simulink model "Furuta_Control"  (R2017a)
settings: Solver=FixedStepAuto  StartTime=0.0  StopTime=10  FixedStep=Ts  RelTol=1e-3
PreLoadFcn:
  | %myBusDef
StartFcn:
  | % Full path to the block
  | %blk = 'Furuta_Control/Bus Creator';
  | 
  | % Attach the event listener
  | %h = add_exec_event_listener(blk, ...
  | %         'PostOutputs', @displayBusdata);
values from neighbouring files (symbols this model uses):
  alpha = J + (M+m1/3+m2)*L1^2    (= 0.00399809399506)    [Furuta_Constants.m]
  beta = (M + m2/3)*L2^2    (= 0.000696322666667)    [Furuta_Constants.m]
  dtDisc = 0.01    [Furuta_Constants.m]
  gamma = (M + m2/2)*L2*L1    (= 0.0006835647)    [Furuta_Constants.m]
  initial_state = pi+15*pi/180    (= 3.40339204139)    [Furuta_Constants.m]
  K = place(Ap,Bp,[-7 -5 -4+4j -4-4j])    [Furuta_Constants.m]
  kb = 2*zeta*omega_n*J    (= 0.000479399222688)    [Furuta_Constants.m]
  ke = 0.182    [Furuta_Constants.m]
  Re = 14.5    [Furuta_Constants.m]
  sigma = (M + m2/2)*g*L2    (= 0.07018074)    [Furuta_Constants.m]
  Ts = 0.001    [Furuta_Constants.m]
libraries: simulink_extras x1, dspinverses x1, sharedTrackingLibrary x1
settings Model: Creator=Marcelo  LastModifiedBy=felip
settings SolverCC: ZeroCrossControl=DisableAll
settings DebuggingCC: ParameterOverflowMsg=warning  BusObjectLabelMismatch=error
settings ModelReferenceCC: ModelReferenceMinAlgLoopOccurrences=on
settings ConfigComp: PLC_TargetIDE=codesys23  PLC_GenerateReport=off

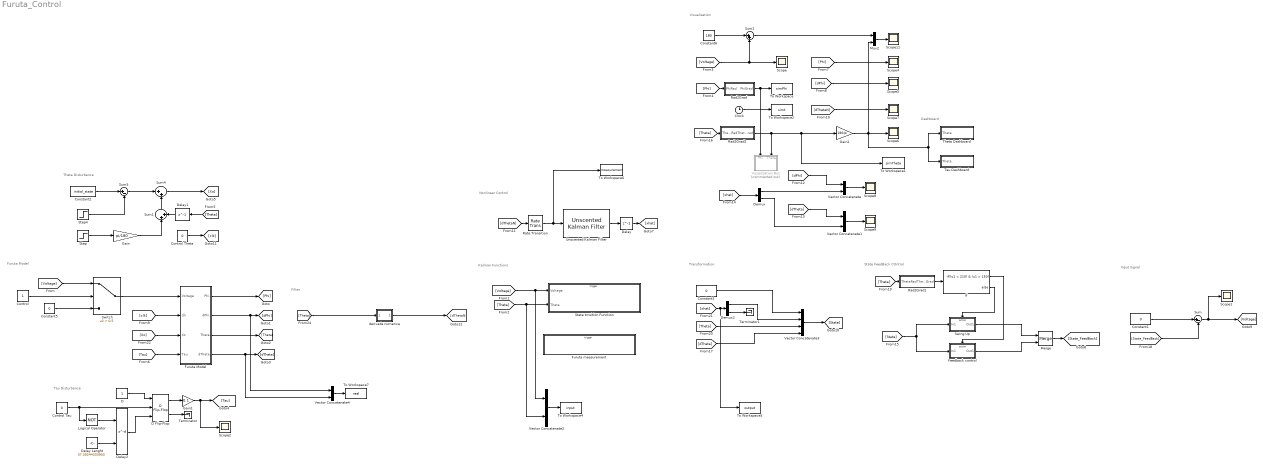
== system Furuta_Control ==
  note: Filter
  note: Tau Disturbance
  note: Dashboard
  note: Theta Disturbance
  note: Transformation
  note: State FeedBack COntrol
  note: Input Signal
  note: Furuta Model
  note: Visualisation
  note: Kalman Functions
  note: Nonlinear Control
  Clock : Clock
  Constant1 : Constant  Value=0
  Constant2 : Constant  Value=initial_state
  Constant3 : Constant  Value=0
  Constant5 : Constant  Value=0
  Constant6 : Constant  Value=180
  Control : Constant
  "Control Tau " : Constant  Value=0  OutDataTypeStr=boolean
  Control Theta : Constant  Value=0
  D : Constant  OutDataTypeStr=boolean
  D Flip-Flop : simulink_extras/Flip Flops/D Flip-Flop
      settings: SourceProductName=Simulink
  Delay : Delay  DelayLength=1  InitialCondition=0
  Delay Lenght : Constant  Value=37.39244333903
  Delay1 : Delay  DelayLength=1
  Delay2 : Delay  DelayLengthSource=Input port
      settings: InputPortMap=u0,p1
  Demux : Demux  Outputs=2
  Demux2 : Demux  Outputs=2
  Feedback control : Subsystem  TreatAsAtomicUnit=on
  "Furuta Model " : Subsystem
  "Furuta measurement " : Subsystem  TreatAsAtomicUnit=on
  Gain : Gain  Gain=pi/180
  Gain1 : Gain  Gain=0.1
  Gain2 : Gain  Gain=180/pi
  If : If  IfExpression=(u1 < 210) & (u1 > 150)
  Logical Operator : Logic  Operator=NOT  AllPortsSameDT=off  OutDataTypeStr=boolean
  Merge : Merge
  Mux2 : Mux  Inputs=2
  Rad2Grad : Subsystem
  Rad2Grad1 : Subsystem
  Rad2Grad2 : Subsystem
  Rate Transition : RateTransition  OutPortSampleTimeOpt=Inherit  OutPortSampleTime=Ts
  Scope{,1..2,4..9,11} (10 alike) : Scope
  "State trnsition Function " : Subsystem  TreatAsAtomicUnit=on
  Step : Step  After=-13.91193695068  SampleTime=0
  Step4 : Step  Time=0.5  After=initial_state  SampleTime=0
  Sum : Sum  Inputs=|+-
  Sum1 : Sum  Inputs=|++
  Sum2 : Sum  Inputs=|++
  Sum4 : Sum  Inputs=|++
  Sum5 : Sum  Inputs=|+-
  Swing Up : Subsystem  TreatAsAtomicUnit=on
  Switch : Switch  Criteria=u2 > Threshold  Threshold=0.5
  Tau Dashboard : Subsystem
  Terminator : Terminator
  Terminator1 : Terminator
  Theta Dashboard : Subsystem
  To Workspace : ToWorkspace  VariableName=simPhi  SampleTime=-1
      settings: Save2DSignal=2-D array (concatenate along first dimension)
  To Workspace1 : ToWorkspace  VariableName=simTheta  SampleTime=-1
      settings: Save2DSignal=2-D array (concatenate along first dimension)
  To Workspace2 : ToWorkspace  VariableName=simt  SampleTime=-1
      settings: Save2DSignal=2-D array (concatenate along first dimension)
  To Workspace4 : ToWorkspace  VariableName=input  SampleTime=-1
      settings: Save2DSignal=2-D array (concatenate along first dimension)
  To Workspace5 : ToWorkspace  VariableName=output  SampleTime=-1
      settings: Save2DSignal=2-D array (concatenate along first dimension)
  To Workspace6 : ToWorkspace  VariableName=measurement  SampleTime=-1
      settings: Save2DSignal=2-D array (concatenate along first dimension)
  To Workspace7 : ToWorkspace  VariableName=real  SampleTime=-1
      settings: Save2DSignal=2-D array (concatenate along first dimension)
  Unscented Kalman Filter : sharedTrackingLibrary/Unscented Kalman Filter  StateTransitionFcn=Furuta_State_Transition  HasAdditiveProcessNoise=Additive  ProcessNoise=diag([2e-8,2e-8])  HasTimeVaryingProcessNoise=off  HasStateTransitionFcnExtraArgument=0  InitialState=[0;0]  InitialStateCovariance=diag([0.001,0.001])  Alpha=1  Beta=2  Kappa=0  MeasurementFcn1=Furuta_Measurement  HasMeasurementEnablePort1=off  HasAdditiveMeasurementNoise1=Additive  MeasurementNoise1=2e-8  HasTimeVaryingMeasurementNoise1=off  HasMeasurementFcnExtraArgument1=0  MeasurementFcn2=myMeasurementFcn  HasMeasurementEnablePort2=off  HasAdditiveMeasurementNoise2=Additive  MeasurementNoise2=1  HasTimeVaryingMeasurementNoise2=off  HasMeasurementFcnExtraArgument2=0  MeasurementFcn3=myMeasurementFcn  HasMeasurementEnablePort3=off  HasAdditiveMeasurementNoise3=Additive  MeasurementNoise3=1  HasTimeVaryingMeasurementNoise3=off  HasMeasurementFcnExtraArgument3=0  MeasurementFcn4=myMeasurementFcn  HasMeasurementEnablePort4=off  HasAdditiveMeasurementNoise4=Additive  MeasurementNoise4=1  HasTimeVaryingMeasurementNoise4=off  HasMeasurementFcnExtraArgument4=0  MeasurementFcn5=myMeasurementFcn  HasMeasurementEnablePort5=off  HasAdditiveMeasurementNoise5=Additive  MeasurementNoise5=1  HasTimeVaryingMeasurementNoise5=off  HasMeasurementFcnExtraArgument5=0  EnableMultirate=off  StateTransitionFcnSampleTime=1  MeasurementFcn1SampleTime=1  MeasurementFcn2SampleTime=1  MeasurementFcn3SampleTime=1  MeasurementFcn4SampleTime=1  MeasurementFcn5SampleTime=1  UseCurrentEstimator=on  OutputStateCovariance=off  DataType=double  SampleTime=Ts  NumberOfMeasurements=1
  Vector Concatenate{,1..2,4} (4 alike) : Concatenate
  Vector Concatenate3 : Concatenate  NumInputs=4
  Visualization Bus : Subsystem  Commented=on
  derivada numerica : Subsystem
  wires:
  "Furuta Model "/1(Phi.) -> [Phi]
  "Furuta Model "/2(dPhi.) -> [dPhi], Vector Concatenate4/1
  [Voltage] -> Sum2/2, Scope/1
  [Phi] -> Scope4/1
  [dPhi] -> Scope5/1
  [dThetaN] -> Scope7/1
  Vector Concatenate/1 -> Scope8/1
  [dPhi] -> Vector Concatenate/1
  Vector Concatenate1/1 -> Scope9/1
  [dTheta] -> Vector Concatenate1/1
  [xhat] -> Demux/1
  Demux/1 -> Vector Concatenate/2
  Demux/2 -> Vector Concatenate1/2
  [dThetaN] -> Rate Transition/1
  Constant1/1 -> Sum/1
  [State_FeedBack] -> Sum/2
  Sum/1 -> Scope1/1, [Voltage]
  Unscented Kalman Filter/1 -> Delay/1
  Delay/1 -> [xhat]
  Demux2/2 -> Terminator1/1
  [xhat] -> To Workspace5/1, Demux2/1
  Vector Concatenate3/1 -> [State]
  Demux2/1 -> Vector Concatenate3/2
  Constant3/1 -> Vector Concatenate3/1
  [Theta] -> Vector Concatenate3/3
  Rad2Grad2/1(ThetaGrad) -> To Workspace1/1, Gain2/1, Visualization Bus/2(Theta)
  Clock/1 -> To Workspace2/1
  Rad2Grad/1(PhiGrad) -> To Workspace/1, Visualization Bus/1(Phi)
  If/2 -> Swing Up/Action
  [State] -> Feedback control/1(In1), Swing Up/1(In1)
  Swing Up/1(Out1) -> Merge/1
  Merge/1 -> [State_FeedBack]
  If/1 -> Feedback control/Action
  Gain2/1 -> Scope6/1, Tau Dashboard/1("Theta "), Theta Dashboard/1(Theta), Mux2/2
  Rad2Grad1/1(ThetaGrad) -> If/1
  [Theta] -> Rad2Grad1/1(ThetaRad)
  "Furuta Model "/4(dTheta.) -> Vector Concatenate4/2, [dTheta]
  [dTheta] -> Vector Concatenate3/4
  Feedback control/1(Out1) -> Merge/2
  Step4/1 -> Sum5/2
  Sum4/1 -> [Xo]
  Sum5/1 -> Sum4/1
  Constant2/1 -> Sum5/1
  Step/1 -> Gain/1
  [Xo] -> "Furuta Model "/3(Xo)
  [clk] -> "Furuta Model "/2("clk ")
  [Voltage] -> Switch/1
  Switch/1 -> "Furuta Model "/1("Voltage ")
  Control/1 -> Switch/2
  Constant5/1 -> Switch/3
  Control Theta/1 -> [clk]
  Sum1/1 -> Sum4/2
  Gain/1 -> Sum1/1
  [Theta] -> Delay1/1
  Delay1/1 -> Sum1/2
  D/1 -> D Flip-Flop/1
  Delay2/1 -> D Flip-Flop/3
  Logical Operator/1 -> Delay2/1
  "Control Tau "/1 -> Logical Operator/1, D Flip-Flop/2
  D Flip-Flop/1 -> Gain1/1
  Gain1/1 -> Scope2/1, [Tau]
  [Tau] -> "Furuta Model "/4(Tau)
  D Flip-Flop/2 -> Terminator/1
  Delay Lenght/1 -> Delay2/2
  [Phi] -> Rad2Grad/1(PhiRad)
  [Theta] -> Rad2Grad2/1(ThetaRad)
  Constant6/1 -> Sum2/1
  Mux2/1 -> Scope11/1
  Sum2/1 -> Mux2/1
  "Furuta Model "/3(Theta.) -> [Theta]
  derivada numerica/1(Out1) -> [dThetaN]
  [Theta] -> derivada numerica/1(In1)
  [Voltage] -> Vector Concatenate2/1, "State trnsition Function "/1("Voltage ")
  [Theta] -> Vector Concatenate2/2, "State trnsition Function "/2("Theta ")
  Vector Concatenate2/1 -> To Workspace4/1
  Vector Concatenate4/1 -> To Workspace7/1
  Rate Transition/1 -> To Workspace6/1, Unscented Kalman Filter/1

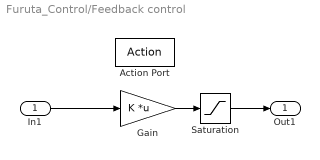
== system Furuta_Control/Feedback control ==
  In1 : Inport
  Action Port : ActionPort  ActionType=then
  Gain : Gain  Gain=K  Multiplication=Matrix(K*u)  ParamDataTypeStr=double  OutDataTypeStr=double
  Saturation : Saturate  UpperLimit=12  LowerLimit=-12
  Out1 : Outport
  wires:
  In1/1 -> Gain/1
  Gain/1 -> Saturation/1
  Saturation/1 -> Out1/1

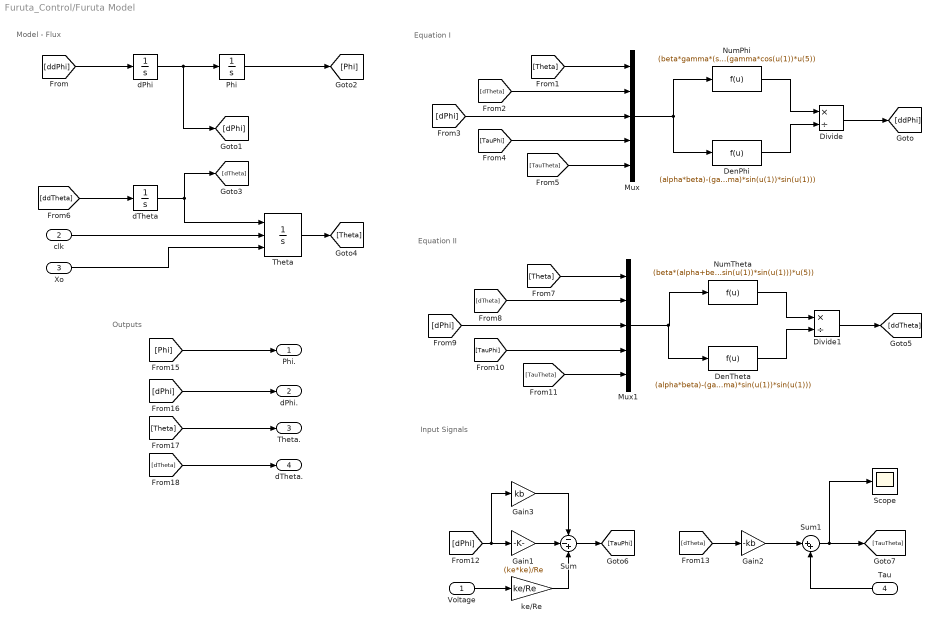
== system Furuta_Control/Furuta Model  ==
  note: Outputs
  note: Input Signals
  note: Equation II
  note: Equation I
  note: Model - Flux
  "Voltage " : Inport
  "clk " : Inport  Port=2
  Xo : Inport  Port=3
  Tau : Inport  Port=4
  DenPhi : Fcn  Expr=(alpha*beta)-(gamma*gamma)+((beta*beta+gamma*gamma)*sin(u(1))*sin(u(1)))
  DenTheta : Fcn  Expr=(alpha*beta)-(gamma*gamma)+((beta*beta+gamma*gamma)*sin(u(1))*sin(u(1)))
  Divide : Product  Inputs=*/
  Divide1 : Product  Inputs=*/
  Gain1 : Gain  Gain=(ke*ke)/Re
  Gain2 : Gain  Gain=-kb
  Gain3 : Gain  Gain=kb
  Mux : Mux  Inputs=5
  Mux1 : Mux  Inputs=5
  NumPhi : Fcn  Expr=(beta*gamma*(sin(u(1))*sin(u(1))-1)*sin(u(1))*u(3)*u(3))-(2*beta*beta*cos(u(1))*sin(u(1))*u(3)*u(2))+(beta*gamma*sin(u(1))*u(2)*u(2))-(gamma*sigma*cos(u(1))*sin(u(1)))+(beta*u(4))-(gamma*cos(u(1))*u(5))
  NumTheta : Fcn  Expr=(beta*(alpha+beta*sin(u(1))*sin(u(1)))*cos(u(1))*sin(u(1))*u(3)*u(3))+(2*beta*gamma*(1-sin(u(1))*sin(u(1)))*sin(u(1))*u(3)*u(2))-(gamma*gamma*cos(u(1))*sin(u(1))*u(2)*u(2))+(sigma*(alpha+beta*sin(u(1))*sin(u(1)))*sin(u(1)))-(gamma*cos(u(1))*u(4))+((alpha+beta*sin(u(1))*sin(u(1)))*u(5))
  Phi : Integrator
  Scope : Scope
  Sum : Sum  Inputs=--+
  Sum1 : Sum  Inputs=|++
  Theta : Integrator  ExternalReset=rising  InitialConditionSource=external  InitialCondition=initial_state
  dPhi : Integrator
  dTheta : Integrator
  "ke/Re " : Gain  Gain=ke/Re
  Phi. : Outport
  dPhi. : Outport  Port=2
  Theta. : Outport  Port=3
  dTheta. : Outport  Port=4
  wires:
  Divide/1 -> [ddPhi]
  "ke/Re "/1 -> Sum/3
  Sum/1 -> [TauPhi]
  Gain1/1 -> Sum/2
  "Voltage "/1 -> "ke/Re "/1
  [dTheta] -> Gain2/1
  Gain3/1 -> Sum/1
  dTheta/1 -> [dTheta], Theta/1
  Theta/1 -> [Theta]
  [Theta] -> Mux1/1
  Mux1/1 -> DenTheta/1, NumTheta/1
  [dTheta] -> Mux1/2
  [dPhi] -> Mux1/3
  [TauTheta] -> Mux1/5
  [TauPhi] -> Mux1/4
  [Theta] -> Mux/1
  [TauTheta] -> Mux/5
  [TauPhi] -> Mux/4
  Phi/1 -> [Phi]
  [dPhi] -> Mux/3
  DenPhi/1 -> Divide/2
  [ddPhi] -> dPhi/1
  [ddTheta] -> dTheta/1
  dPhi/1 -> [dPhi], Phi/1
  NumTheta/1 -> Divide1/1
  NumPhi/1 -> Divide/1
  DenTheta/1 -> Divide1/2
  Mux/1 -> DenPhi/1, NumPhi/1
  [dPhi] -> Gain3/1, Gain1/1
  [dTheta] -> Mux/2
  Divide1/1 -> [ddTheta]
  [Phi] -> Phi./1
  [dPhi] -> dPhi./1
  [Theta] -> Theta./1
  [dTheta] -> dTheta./1
  "clk "/1 -> Theta/2
  Xo/1 -> Theta/3
  Gain2/1 -> Sum1/1
  Sum1/1 -> Scope/1, [TauTheta]
  Tau/1 -> Sum1/2

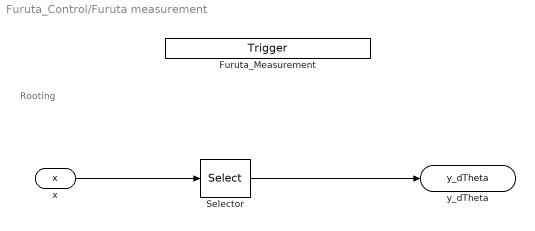
== system Furuta_Control/Furuta measurement  ==
  note: Rooting
  Furuta_Measurement : TriggerPort  TriggerType=function-call  IsSimulinkFunction=on  FunctionName=Furuta_Measurement  VariantControl=Variant
  Selector : Selector  InputPortWidth=2  IndexOptions=Index vector (dialog)  Indices=2  OutputSizes=1
  x : ArgIn  DisableCoverage=on  PortDimensions=2  ArgumentName=x
  y_dTheta : ArgOut  DisableCoverage=on  ArgumentName=y_dTheta
  wires:
  x/1 -> Selector/1
  Selector/1 -> y_dTheta/1

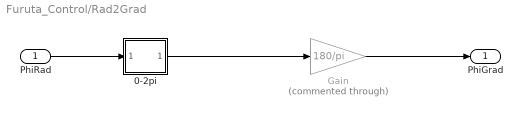
== system Furuta_Control/Rad2Grad ==
  PhiRad : Inport
  0-2pi : Subsystem
  Gain : Gain  Commented=through  Gain=180/pi
  PhiGrad : Outport
  wires:
  0-2pi/1(Out1) -> Gain/1
  Gain/1 -> PhiGrad/1
  PhiRad/1 -> 0-2pi/1(In1)

== system Furuta_Control/Rad2Grad1 ==
  ThetaRad : Inport
  0-2pi : Subsystem
  Gain2 : Gain  Gain=180/pi
  ThetaGrad : Outport
  wires:
  ThetaRad/1 -> 0-2pi/1(In1)
  0-2pi/1(Out1) -> Gain2/1
  Gain2/1 -> ThetaGrad/1

== system Furuta_Control/Rad2Grad2 ==
  ThetaRad : Inport
  0-2pi : Subsystem
  ThetaGrad : Outport
  wires:
  ThetaRad/1 -> 0-2pi/1(In1)
  0-2pi/1(Out1) -> ThetaGrad/1

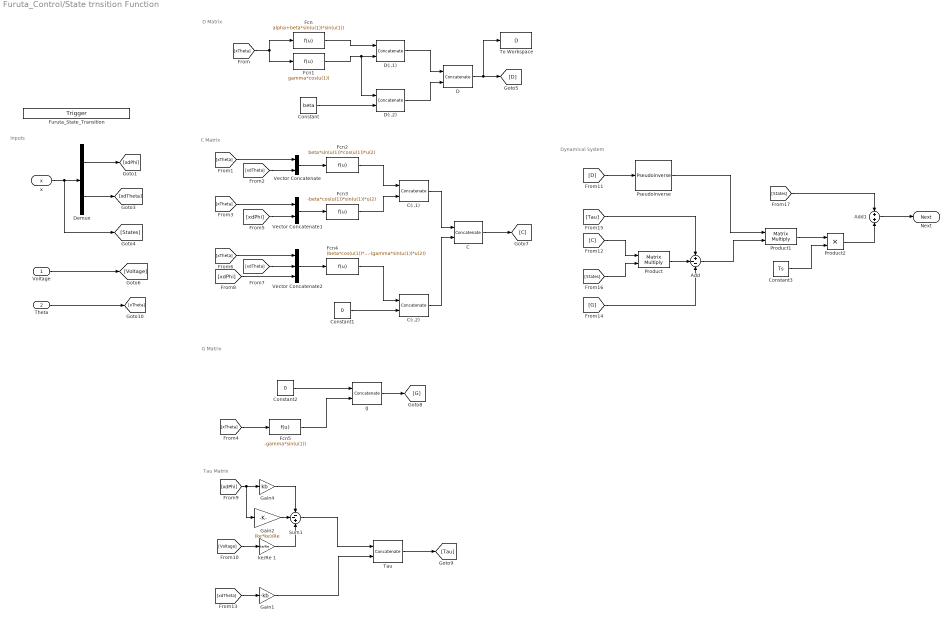
== system Furuta_Control/State trnsition Function  ==
  note: Dynamical System
  note: Tau Matrix
  note: G Matrix
  note: Inputs
  note: D Matrix
  note: C Matrix
  "Voltage " : Inport
  "Theta " : Inport  Port=2
  Furuta_State_Transition : TriggerPort  TriggerType=function-call  IsSimulinkFunction=on  FunctionName=Furuta_State_Transition  VariantControl=Variant
  Add : Sum  Inputs=+--
  Add1 : Sum
  C : Concatenate  Mode=Multidimensional array  ConcatenateDimension=2
  C(:,1) : Concatenate  ConcatenateDimension=2
  C(:,2) : Concatenate  ConcatenateDimension=2
  Constant : Constant  Value=beta
  Constant1 : Constant  Value=0
  Constant2 : Constant  Value=0
  Constant3 : Constant  Value=Ts
  D : Concatenate  Mode=Multidimensional array  ConcatenateDimension=2
  "D(:,1) " : Concatenate  ConcatenateDimension=2
  D(:,2) : Concatenate  ConcatenateDimension=2
  Demux : Demux  Outputs=2
  Fcn : Fcn  Expr=alpha+beta*sin(u(1))*sin(u(1))
  Fcn1 : Fcn  Expr=gamma*cos(u(1))
  Fcn2 : Fcn  Expr=beta*sin(u(1))*cos(u(1))*u(2)
  Fcn3 : Fcn  Expr=-beta*cos(u(1))*sin(u(1))*u(2)
  Fcn4 : Fcn  Expr=(beta*cos(u(1))*sin(u(1))*u(3))-(gamma*sin(u(1))*u(2))
  Fcn5 : Fcn  Expr=-gamma*sin(u(1))
  Gain1 : Gain  Gain=-kb
  Gain2 : Gain  Gain=(ke*ke)/Re
  Gain4 : Gain  Gain=kb
  Product : Product  Multiplication=Matrix(*)
  Product1 : Product  Multiplication=Matrix(*)
  Product2 : Product
  Pseudoinverse : dspinverses/Pseudoinverse  wanterr=off  SimulateUsing=Interpreted execution
      settings: SourceProductName=DSP System Toolbox  SourceProductBaseCode=DS
  Sum1 : Sum  Inputs=--+
  Tau : Concatenate  ConcatenateDimension=2
  To Workspace : ToWorkspace  VariableName=D  SampleTime=-1
  Vector Concatenate : Concatenate
  Vector Concatenate1 : Concatenate
  Vector Concatenate2 : Concatenate  NumInputs=3
  g : Concatenate  ConcatenateDimension=2
  ke/Re 1 : Gain  Gain=ke/Re
  x : ArgIn  DisableCoverage=on  PortDimensions=2  ArgumentName=x
      settings: LockScale=on
  Next : ArgOut  DisableCoverage=on  PortDimensions=2  ArgumentName=Next
  wires:
  x/1 -> [States], Demux/1
  Demux/2 -> [xdTheta]
  "D(:,1) "/1 -> D/1
  D(:,2)/1 -> D/2
  Fcn/1 -> "D(:,1) "/1
  Fcn1/1 -> "D(:,1) "/2, D(:,2)/1
  [xTheta] -> Fcn/1, Fcn1/1
  Constant/1 -> D(:,2)/2
  Fcn3/1 -> C(:,1)/2
  Constant1/1 -> C(:,2)/2
  C(:,2)/1 -> C/2
  Fcn2/1 -> C(:,1)/1
  C(:,1)/1 -> C/1
  Vector Concatenate/1 -> Fcn2/1
  [xTheta] -> Vector Concatenate/1
  [xdTheta] -> Vector Concatenate/2
  Vector Concatenate1/1 -> Fcn3/1
  [xTheta] -> Vector Concatenate1/1
  [xdPhi] -> Vector Concatenate2/3
  Fcn4/1 -> C(:,2)/1
  Vector Concatenate2/1 -> Fcn4/1
  [xdTheta] -> Vector Concatenate2/2
  [xTheta] -> Vector Concatenate2/1
  [xdPhi] -> Vector Concatenate1/2
  Constant2/1 -> g/1
  [xTheta] -> Fcn5/1
  Fcn5/1 -> g/2
  Gain2/1 -> Sum1/2
  Gain4/1 -> Sum1/1
  [xdPhi] -> Gain2/1, Gain4/1
  ke/Re 1/1 -> Sum1/3
  [Voltage] -> ke/Re 1/1
  "Voltage "/1 -> [Voltage]
  Sum1/1 -> Tau/1
  Gain1/1 -> Tau/2
  [xdTheta] -> Gain1/1
  D/1 -> To Workspace/1, [D]
  C/1 -> [C]
  g/1 -> [G]
  Tau/1 -> [Tau]
  [D] -> Pseudoinverse/1
  [States] -> Product/2
  [C] -> Product/1
  [Tau] -> Add/1
  Product/1 -> Add/2
  [G] -> Add/3
  Add/1 -> Product1/2
  Pseudoinverse/1 -> Product1/1
  Add1/1 -> Next/1
  Product1/1 -> Product2/1
  Constant3/1 -> Product2/2
  Product2/1 -> Add1/2
  [States] -> Add1/1
  Demux/1 -> [xdPhi]
  "Theta "/1 -> [xTheta]

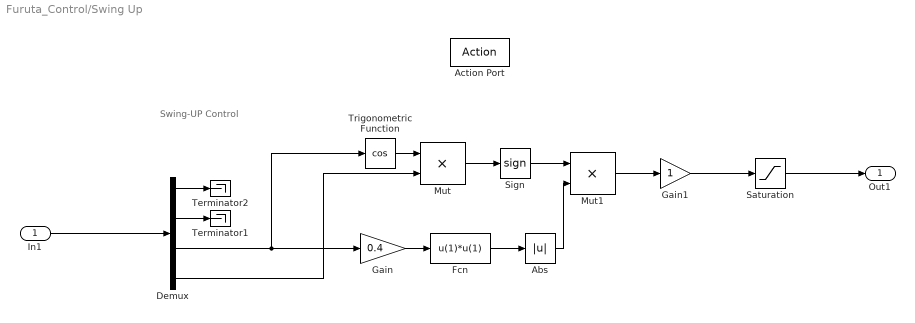
== system Furuta_Control/Swing Up ==
  note: Swing-UP Control
  In1 : Inport
  Action Port : ActionPort  ActionType=else
  Abs : Abs
  Demux : Demux
  Fcn : Fcn  Expr=u(1)*u(1)
  Gain : Gain  Gain=0.4
  Gain1 : Gain
  Mut : Product  Inputs=**
  Mut1 : Product  Inputs=**
  Saturation : Saturate  UpperLimit=12  LowerLimit=-12
  Sign : Signum
  Terminator1 : Terminator
  Terminator2 : Terminator
  Trigonometric Function : Trigonometry  Operator=cos
  Out1 : Outport  InitialOutput=0
  wires:
  Saturation/1 -> Out1/1
  Demux/2 -> Terminator1/1
  Demux/1 -> Terminator2/1
  Gain1/1 -> Saturation/1
  Mut1/1 -> Gain1/1
  Demux/3 -> Trigonometric Function/1, Gain/1
  Fcn/1 -> Abs/1
  Trigonometric Function/1 -> Mut/1
  Demux/4 -> Mut/2
  Abs/1 -> Mut1/2
  Sign/1 -> Mut1/1
  Mut/1 -> Sign/1
  Gain/1 -> Fcn/1
  In1/1 -> Demux/1

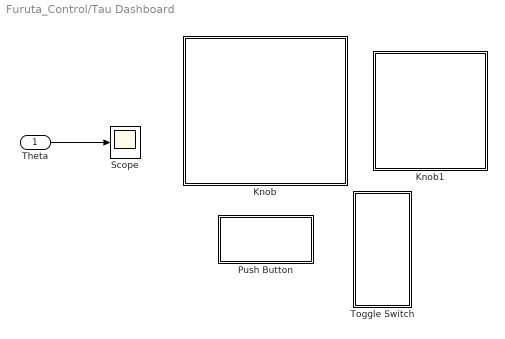
== system Furuta_Control/Tau Dashboard ==
  "Theta " : Inport
  Knob : Subsystem  DialogController=hmiCreateDDGDialog  IsWebBlock=on  mask(MWDashboardBlock){webBlockId=4df3a667-03b8-4ac4-b39a-9a126b51fd8c, webBlockType=continuousknob, ShowInLibBrowser=on, ShowInitialText=on, HMISrcModelName=Furuta_Control}
      mask prompts: webBlockId "WebBlock Id"; webBlockType "WebBlock Type"; HMISrcModelName "Source Model"
      mask help: SimulinkHMI:dialogs:ContinuousKnobDialogDesc
      mask Help: helpview([docroot '/mapfiles/simulink.map'], 'hmi_knob')
      mask Display:
      | if strcmp(get_param(bdroot(gcb),'BlockDiagramType'), 'library')
      |     image([(matlabroot) '/toolbox/simulink/hmi/icons/ContinuousKnob.png']);
      | end
  Knob1 : Subsystem  DialogController=hmiCreateDDGDialog  IsWebBlock=on  mask(MWDashboardBlock){webBlockId=2ffdbfce-ad2c-4f82-8aaa-bb0c61bbc096, webBlockType=continuousknob, ShowInLibBrowser=on, ShowInitialText=on, HMISrcModelName=Furuta_Control}
      mask prompts: webBlockId "WebBlock Id"; webBlockType "WebBlock Type"; HMISrcModelName "Source Model"
      mask help: SimulinkHMI:dialogs:ContinuousKnobDialogDesc
      mask Help: helpview([docroot '/mapfiles/simulink.map'], 'hmi_knob')
      mask Display:
      | if strcmp(get_param(bdroot(gcb),'BlockDiagramType'), 'library')
      |     image([(matlabroot) '/toolbox/simulink/hmi/icons/ContinuousKnob.png']);
      | end
  Push Button : Subsystem  DialogController=hmiCreateDDGDialog  IsWebBlock=on  mask(MWDashboardBlock){webBlockId=54a9afda-0d0c-4fe3-9fd9-a5fd5bfd2eff, webBlockType=pushbutton, ShowInLibBrwoser=on, ShowInitialText=on, HMISrcModelName=Furuta_Control}
      mask prompts: webBlockId "WebBlock Id"; webBlockType "WebBlock Type"; HMISrcModelName "Source Model"
      mask help: SimulinkHMI:dialogs:PushButtonDialogDesc
      mask Help: helpview([docroot '/mapfiles/simulink.map'], 'hmi_push_button')
      mask Display:
      | model = bdroot(gcb);
      | if strcmp(get_param(model,'BlockDiagramType'), 'library')
      |     image([(matlabroot) '/toolbox/simulink/hmi/icons/PushButton.png']);
      | end
  Scope : Scope
  Toggle Switch : Subsystem  DialogController=hmiCreateDDGDialog  IsWebBlock=on  mask(MWDashboardBlock){webBlockId=9ef78f83-ce25-4a6d-8579-1dd4683104fe, webBlockType=toggleswitch, ShowInLibBrowser=on, ShowInitialText=on, HMISrcModelName=Furuta_Control}
      mask prompts: webBlockId "WebBlock Id"; webBlockType "WebBlock Type"; HMISrcModelName "Source Model"
      mask help: SimulinkHMI:dialogs:SwitchDialogDesc
      mask Help: helpview([docroot '/mapfiles/simulink.map'], 'hmi_toggle_switch')
      mask Display:
      | if strcmp(get_param(bdroot(gcb),'BlockDiagramType'), 'library')
      |     image([(matlabroot) '/toolbox/simulink/hmi/icons/ToggleSwitch.png']);
      | end
  wires:
  "Theta "/1 -> Scope/1

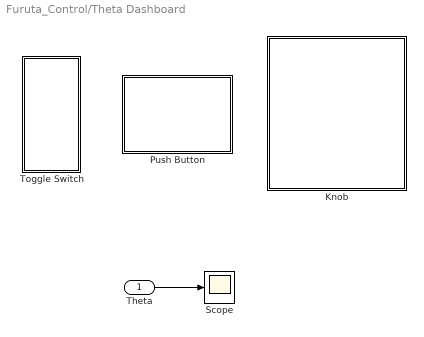
== system Furuta_Control/Theta Dashboard ==
  Theta : Inport
  Knob : Subsystem  DialogController=hmiCreateDDGDialog  IsWebBlock=on  mask(MWDashboardBlock){webBlockId=aac29083-8fd0-4520-b4bd-68fb2bedaac5, webBlockType=continuousknob, ShowInLibBrowser=on, ShowInitialText=on, HMISrcModelName=Furuta_Control}
      mask prompts: webBlockId "WebBlock Id"; webBlockType "WebBlock Type"; HMISrcModelName "Source Model"
      mask help: SimulinkHMI:dialogs:ContinuousKnobDialogDesc
      mask Help: helpview([docroot '/mapfiles/simulink.map'], 'hmi_knob')
      mask Display:
      | if strcmp(get_param(bdroot(gcb),'BlockDiagramType'), 'library')
      |     image([(matlabroot) '/toolbox/simulink/hmi/icons/ContinuousKnob.png']);
      | end
  Push Button : Subsystem  DialogController=hmiCreateDDGDialog  IsWebBlock=on  mask(MWDashboardBlock){webBlockId=316806c3-a7e8-4532-a90d-ebec42bbe281, webBlockType=pushbutton, ShowInLibBrwoser=on, ShowInitialText=on, HMISrcModelName=Furuta_Control}
      mask prompts: webBlockId "WebBlock Id"; webBlockType "WebBlock Type"; HMISrcModelName "Source Model"
      mask help: SimulinkHMI:dialogs:PushButtonDialogDesc
      mask Help: helpview([docroot '/mapfiles/simulink.map'], 'hmi_push_button')
      mask Display:
      | model = bdroot(gcb);
      | if strcmp(get_param(model,'BlockDiagramType'), 'library')
      |     image([(matlabroot) '/toolbox/simulink/hmi/icons/PushButton.png']);
      | end
  Scope : Scope
  Toggle Switch : Subsystem  DialogController=hmiCreateDDGDialog  IsWebBlock=on  mask(MWDashboardBlock){webBlockId=1ab1796d-89f8-4362-a8ce-2d672f8a6157, webBlockType=toggleswitch, ShowInLibBrowser=on, ShowInitialText=on, HMISrcModelName=Furuta_Control}
      mask prompts: webBlockId "WebBlock Id"; webBlockType "WebBlock Type"; HMISrcModelName "Source Model"
      mask help: SimulinkHMI:dialogs:SwitchDialogDesc
      mask Help: helpview([docroot '/mapfiles/simulink.map'], 'hmi_toggle_switch')
      mask Display:
      | if strcmp(get_param(bdroot(gcb),'BlockDiagramType'), 'library')
      |     image([(matlabroot) '/toolbox/simulink/hmi/icons/ToggleSwitch.png']);
      | end
  wires:
  Theta/1 -> Scope/1

== system Furuta_Control/Visualization Bus ==
  Phi : Inport
  Theta : Inport  Port=2
  Bus Creator : BusCreator  Inputs=2  OutDataTypeStr=Bus: BO  NonVirtualBus=on
  Terminator : Terminator
  wires:
  Theta/1 -> Bus Creator/2
  Phi/1 -> Bus Creator/1
  Bus Creator/1 -> Terminator/1

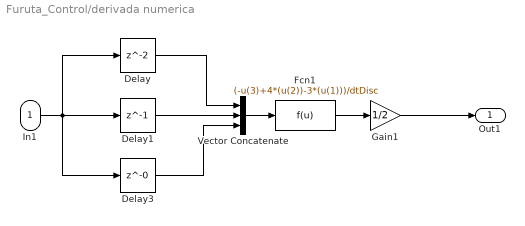
== system Furuta_Control/derivada numerica ==
  In1 : Inport
  Delay : Delay  InitialCondition=0  SampleTime=dtDisc
  Delay1 : Delay  DelayLength=1  InitialCondition=0  SampleTime=dtDisc
  Delay3 : Delay  DelayLength=0  InitialCondition=0  SampleTime=dtDisc
  Fcn1 : Fcn  Expr=(-u(3)+4*(u(2))-3*(u(1)))/dtDisc
  Gain1 : Gain  Gain=1/2
  Vector Concatenate : Concatenate  NumInputs=3
  Out1 : Outport
  wires:
  Fcn1/1 -> Gain1/1
  Delay1/1 -> Vector Concatenate/2
  Vector Concatenate/1 -> Fcn1/1
  Delay/1 -> Vector Concatenate/1
  Delay3/1 -> Vector Concatenate/3
  Gain1/1 -> Out1/1
  In1/1 -> Delay1/1, Delay/1, Delay3/1

== system Furuta_Control/Rad2Grad/0-2pi ==
  In1 : Inport
  2pi : Constant  Value=2*pi
  Math Function : Math  Operator=mod  SaturateOnIntegerOverflow=on
  Out1 : Outport
  wires:
  2pi/1 -> Math Function/2
  Math Function/1 -> Out1/1
  In1/1 -> Math Function/1

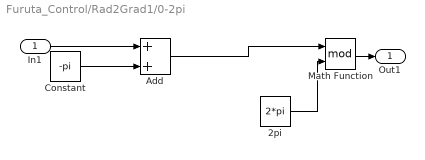
== system Furuta_Control/Rad2Grad1/0-2pi ==
  In1 : Inport
  2pi : Constant  Value=2*pi
  Add : Sum
  Constant : Constant  Value=-pi
  Math Function : Math  Operator=mod  SaturateOnIntegerOverflow=on
  Out1 : Outport
  wires:
  Math Function/1 -> Out1/1
  2pi/1 -> Math Function/2
  Constant/1 -> Add/2
  In1/1 -> Add/1
  Add/1 -> Math Function/1

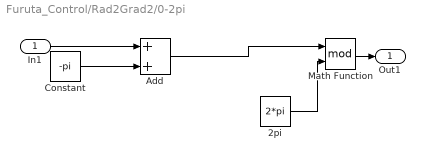
== system Furuta_Control/Rad2Grad2/0-2pi ==
  In1 : Inport
  2pi : Constant  Value=2*pi
  Add : Sum
  Constant : Constant  Value=-pi
  Math Function : Math  Operator=mod  SaturateOnIntegerOverflow=on
  Out1 : Outport
  wires:
  Math Function/1 -> Out1/1
  2pi/1 -> Math Function/2
  Constant/1 -> Add/2
  In1/1 -> Add/1
  Add/1 -> Math Function/1

== system Furuta_Control/Tau Dashboard/Knob ==

== system Furuta_Control/Tau Dashboard/Knob1 ==

== system Furuta_Control/Tau Dashboard/Push Button ==

== system Furuta_Control/Tau Dashboard/Toggle Switch ==

== system Furuta_Control/Theta Dashboard/Knob ==

== system Furuta_Control/Theta Dashboard/Push Button ==

== system Furuta_Control/Theta Dashboard/Toggle Switch ==
